simulink model "SVM_test2"  (R2020a)
(part 4 of 9)

      mask init:
      | % blkh = gcbh;
      | % [sfi, sfp, sfpt] = rti_fpga_blockinitial(blkh,'UPDATEPARAMETER');
      | % rti_fpga_blockinitial(blkh,'UPDATEBLOCKGUI');
      settings: CopyFcn=try, rti_fpga_blk_copyfcn(gcbh); catch,errordlg({lasterr, '','Please check your RTI installation.'},['Error: ' upper(bdroot)], 'replace'); end  DeleteFcn=try, rti_fpga_blk_deletefcn(gcbh); catch,errordlg({lasterr, '','Please check your RTI installation.'},['Error: ' upper(bdroot)], 'replace'); end  ModelCloseFcn=try, rti_fpga_blk_modelclosefcn(gcbh); catch,errordlg({lasterr, '','Please check your RTI installation.'},['Error: ' upper(bdroot)], 'replace'); end  PreSaveFcn=try, rti_fpga_blk_presavefcn(gcbh); catch,errordlg({lasterr, '','Please check your RTI installation.'},['Error: ' upper(bdroot)], 'replace'); end  NameChangeFcn=try, rti_fpga_blk_namechangefcn(gcbh); catch,errordlg({lasterr, '','Please check your RTI installation.'},['Error: ' upper(bdroot)], 'replace'); end  OpenFcn=try, rti_fpga_blk_openfcn(gcbh); catch,errordlg({lasterr, '','Please check your RTI installation.'},['Error: ' upper(bdroot)], 'replace'); end  CloseFcn=try, rti_fpga_blk_closefcn(gcbh); catch,errordlg({lasterr, '','Please check your RTI installation.'},['Error: ' upper(bdroot)], 'replace'); end  ParentCloseFcn=try, rti_fpga_blk_parentclosefcn(gcbh); catch,errordlg({lasterr, '','Please check your RTI installation.'},['Error: ' upper(bdroot)], 'replace'); end
      mask Help: eval( ['lasterror(''reset''); rtifpgaguilib(''RTIMaskHelp'', gcbh);', 'disp(lasterr);']);
      mask Display: text(0.5,0.65,'Register In 3','HorizontalAlignment','center');text(0.5,0.5,'cl','HorizontalAlignment','center');text(0.5,0.35,'Group: 1','HorizontalAlignment','center');
  FPGA_XDATA_READ_BL4 : Subsystem  LoadFcn=try, rti_fpga_blk_loadfcn(gcbh); catch,errordlg({lasterr, '','Please check your RTI installation.'},['Error: ' upper(bdroot)], 'replace'); end  InitFcn=try, rti_fpga_blk_initfcn(gcbh); catch,errordlg({lasterr, '','Please check your RTI installation.'},['Error: ' upper(bdroot)], 'replace'); end  StartFcn=try, rti_fpga_blk_startfcn(gcbh); catch,errordlg({lasterr, '','Please check your RTI installation.'},['Error: ' upper(bdroot)], 'replace'); end  mask(RTI){DSProperties=struct('RTI',struct('Version',uint32(6),'BlockType',struct('isSLSource',uint8(1),'isSLSink',uint8(0),'isHWSource',uint8(0),'isHWSink',uint8(0),'isSetup',uint8(1),'isInline',uint8(1),'isNonInline',uint8(0),'isInterrupt',uint8(0),'isChannelwise',uint8(0)),'IOBoardType','DSFPGA','UnitType','','Identifier','PHSREAD','DialogType','ML','BlockSet','FPGA','SlaveProcessor','')), RTIBlockInterface=struct('OutputPortsActive',1,'OutputPortsWidth',int32(1),'OutputPortsDataType',{{'SS_DOUBLE'}},'OutputPortsName',{{['From XDATA']}},'InitLevel',3,'DialogFcn','rtifpgaphsreadgui','BlockDisplay',{{['XDATA Read'],'auto'}},'IconTransparency','on','BlockName',struct('Token',{{'FPGA_XDATA_Read_BL1'}})), RTIBlockParameters=struct('BoardNo',{{1,'OFF',[1 16]}},'Name',{{['Register In 4'],'OFF',[]}},'CustomName',{{'d1','OFF',[]}},'AccessTyp',{{'Register','OFF',[]}},'ChannelNo',{{'4','OFF',[]}},'FrmIni',{{'fpga_framework_ini_DS1302_XC7K325T_FLEXIBLEIO','OFF',[]}},'DynFcn',{{struct('GUIPar',struct('Name',{{['Binary point position (or fraction width)']},{'Format'},{['Register Group ID']},{['Enable simulation port']},{['Simulation ports sample time']},{['Used Flag']}},'GUIType',{{'edit'},{'popup','signed','unsigned','floating-point'},{'edit'},{'checkbox'},{'edit'},{'none'}},'Range',{{[0 1 2 3 4 5 6 7 8 9 10 11 12 13 14 15 16 17 18 19 20 21 22 23 24 25 26 27 28 29 30 31 32]},{'signed','unsigned','floating-point'},{[0 1 2 3 4 5 6 7 8 9 10 11 12 13 14 15 16 17 18 19 20 21 22 23 24 25 26 27 28 29 30 31 32 33 34 35 36 37 38 39 40 41 42 43 44 45 46 47 48 49 50 51 52 53 54 55 56 57 58 59 60 61 62 63]},{'0','1'},{''},{'0','1'}},'Init',{{'0'},{'signed'},{'0'},{'0'},{'-1','1'},{'1','0'}},'Group',{{''},{''},{''},{''},{''},{''}},'Generic',{{''},{''},{'xreg2fpga_group_003'},{''},{'REGISTER_IN_003_SIM_PORT_SAMPLE_TIME'},{'xreg2fpga_inst_003'}},'Application',{{''},{''},{''},{'ApplicationOut(1).Show'},{''},{''}},'Framework',{{'FrameworkIn(1).BinaryPoint'},{'FrameworkIn(1).Format'},{''},{''},{''},{''}},'Callback',{{'proc_bus_fpga_framework_ini_DS1302:fraction_width'},{'proc_bus_fpga_framework_ini_DS1302:fraction_width'},{''},{''},{''},{''}}),'Exl',{{''}},'HlpFile',{{'rtifpga','REGISTER_IN_DS1302'}},'Hlp',{{['Click below for further details on this I/O function.']}},'Gen',struct('name',{'','','xreg2fpga_group_003','','REGISTER_IN_003_SIM_PORT_SAMPLE_TIME','xreg2fpga_inst_003'},'value',{'','','1','','-1','1'},'unusedinit',{'','','','','1','0'},'tag',{'','','','','',''},'filename',{'','','','','',''}),'Frm',struct('FrameworkOut',struct('Name',{},'BitWidth',{},'BinaryPoint',{},'Format',{}),'FrameworkIn',struct('Name',{{'xreg_003_dout'},{'xreg_003_dout_wr'}},'BitWidth',{{'32'},{'1'}},'BinaryPoint',{{'0'},{'0'}},'Format',{{'unsigned'},{'unsigned'}},'DownSample',{[],{true}})),'App',struct('ApplicationOut',struct('Name',{{'Sim_Data'}},'Show',{{0}}),'ApplicationIn',struct('Name',{{'Data'},{['Data New']}},'Show',{{true},{true}})),'Con',{{'FrameworkIn(1)','ApplicationIn(1)','FrameworkIn(2)','ApplicationIn(2)'}},'OffCon',{{'data_o','FrameworkIn(1)','data_i','ApplicationOut(1)','data_new_o','FrameworkIn(2)'}},'OffModel',{{'phs_read_register'}}),'OFF',[]}},'FPGAFrameworkId',{{'8','OFF',[]}},'BusSettings',{{[' '],'OFF',[]}},'SubChannelNo',{{'1','OFF',[]}}), RTISFcnParameters=struct('BoardNo','double'), RTIBlockParaDefault=struct('BoardNo',1,'Name',[' '],'CustomName',[' '],'AccessTyp',['<not selected>'],'ChannelNo',[' '],'FrmIni',[' '],'DynFcn',struct('GUIPar','','Hlp','','HlpFile','','Frm','','Gen','','Exl','','App','','Con',''),'FPGAFrameworkId',[' '],'BusSettings',[' '],'SubChannelNo','1')}
      mask init:
      | % blkh = gcbh;
      | % [sfi, sfp, sfpt] = rti_fpga_blockinitial(blkh,'UPDATEPARAMETER');
      | % rti_fpga_blockinitial(blkh,'UPDATEBLOCKGUI');
      settings: CopyFcn=try, rti_fpga_blk_copyfcn(gcbh); catch,errordlg({lasterr, '','Please check your RTI installation.'},['Error: ' upper(bdroot)], 'replace'); end  DeleteFcn=try, rti_fpga_blk_deletefcn(gcbh); catch,errordlg({lasterr, '','Please check your RTI installation.'},['Error: ' upper(bdroot)], 'replace'); end  ModelCloseFcn=try, rti_fpga_blk_modelclosefcn(gcbh); catch,errordlg({lasterr, '','Please check your RTI installation.'},['Error: ' upper(bdroot)], 'replace'); end  PreSaveFcn=try, rti_fpga_blk_presavefcn(gcbh); catch,errordlg({lasterr, '','Please check your RTI installation.'},['Error: ' upper(bdroot)], 'replace'); end  NameChangeFcn=try, rti_fpga_blk_namechangefcn(gcbh); catch,errordlg({lasterr, '','Please check your RTI installation.'},['Error: ' upper(bdroot)], 'replace'); end  OpenFcn=try, rti_fpga_blk_openfcn(gcbh); catch,errordlg({lasterr, '','Please check your RTI installation.'},['Error: ' upper(bdroot)], 'replace'); end  CloseFcn=try, rti_fpga_blk_closefcn(gcbh); catch,errordlg({lasterr, '','Please check your RTI installation.'},['Error: ' upper(bdroot)], 'replace'); end  ParentCloseFcn=try, rti_fpga_blk_parentclosefcn(gcbh); catch,errordlg({lasterr, '','Please check your RTI installation.'},['Error: ' upper(bdroot)], 'replace'); end
      mask Help: eval( ['lasterror(''reset''); rtifpgaguilib(''RTIMaskHelp'', gcbh);', 'disp(lasterr);']);
      mask Display: text(0.5,0.65,'Register In 4','HorizontalAlignment','center');text(0.5,0.5,'d1','HorizontalAlignment','center');text(0.5,0.35,'Group: 1','HorizontalAlignment','center');
  FPGA_XDATA_READ_BL5 : Subsystem  LoadFcn=try, rti_fpga_blk_loadfcn(gcbh); catch,errordlg({lasterr, '','Please check your RTI installation.'},['Error: ' upper(bdroot)], 'replace'); end  InitFcn=try, rti_fpga_blk_initfcn(gcbh); catch,errordlg({lasterr, '','Please check your RTI installation.'},['Error: ' upper(bdroot)], 'replace'); end  StartFcn=try, rti_fpga_blk_startfcn(gcbh); catch,errordlg({lasterr, '','Please check your RTI installation.'},['Error: ' upper(bdroot)], 'replace'); end  mask(RTI){DSProperties=struct('RTI',struct('Version',uint32(6),'BlockType',struct('isSLSource',uint8(1),'isSLSink',uint8(0),'isHWSource',uint8(0),'isHWSink',uint8(0),'isSetup',uint8(1),'isInline',uint8(1),'isNonInline',uint8(0),'isInterrupt',uint8(0),'isChannelwise',uint8(0)),'IOBoardType','DSFPGA','UnitType','','Identifier','PHSREAD','DialogType','ML','BlockSet','FPGA','SlaveProcessor','')), RTIBlockInterface=struct('OutputPortsActive',1,'OutputPortsWidth',int32(1),'OutputPortsDataType',{{'SS_DOUBLE'}},'OutputPortsName',{{['From XDATA']}},'InitLevel',3,'DialogFcn','rtifpgaphsreadgui','BlockDisplay',{{['XDATA Read'],'auto'}},'IconTransparency','on','BlockName',struct('Token',{{'FPGA_XDATA_Read_BL1'}})), RTIBlockParameters=struct('BoardNo',{{1,'OFF',[1 16]}},'Name',{{['Register In 5'],'OFF',[]}},'CustomName',{{'d2','OFF',[]}},'AccessTyp',{{'Register','OFF',[]}},'ChannelNo',{{'5','OFF',[]}},'FrmIni',{{'fpga_framework_ini_DS1302_XC7K325T_FLEXIBLEIO','OFF',[]}},'DynFcn',{{struct('GUIPar',struct('Name',{{['Binary point position (or fraction width)']},{'Format'},{['Register Group ID']},{['Enable simulation port']},{['Simulation ports sample time']},{['Used Flag']}},'GUIType',{{'edit'},{'popup','signed','unsigned','floating-point'},{'edit'},{'checkbox'},{'edit'},{'none'}},'Range',{{[0 1 2 3 4 5 6 7 8 9 10 11 12 13 14 15 16 17 18 19 20 21 22 23 24 25 26 27 28 29 30 31 32]},{'signed','unsigned','floating-point'},{[0 1 2 3 4 5 6 7 8 9 10 11 12 13 14 15 16 17 18 19 20 21 22 23 24 25 26 27 28 29 30 31 32 33 34 35 36 37 38 39 40 41 42 43 44 45 46 47 48 49 50 51 52 53 54 55 56 57 58 59 60 61 62 63]},{'0','1'},{''},{'0','1'}},'Init',{{'0'},{'signed'},{'0'},{'0'},{'-1','1'},{'1','0'}},'Group',{{''},{''},{''},{''},{''},{''}},'Generic',{{''},{''},{'xreg2fpga_group_004'},{''},{'REGISTER_IN_004_SIM_PORT_SAMPLE_TIME'},{'xreg2fpga_inst_004'}},'Application',{{''},{''},{''},{'ApplicationOut(1).Show'},{''},{''}},'Framework',{{'FrameworkIn(1).BinaryPoint'},{'FrameworkIn(1).Format'},{''},{''},{''},{''}},'Callback',{{'proc_bus_fpga_framework_ini_DS1302:fraction_width'},{'proc_bus_fpga_framework_ini_DS1302:fraction_width'},{''},{''},{''},{''}}),'Exl',{{''}},'HlpFile',{{'rtifpga','REGISTER_IN_DS1302'}},'Hlp',{{['Click below for further details on this I/O function.']}},'Gen',struct('name',{'','','xreg2fpga_group_004','','REGISTER_IN_004_SIM_PORT_SAMPLE_TIME','xreg2fpga_inst_004'},'value',{'','','1','','-1','1'},'unusedinit',{'','','','','1','0'},'tag',{'','','','','',''},'filename',{'','','','','',''}),'Frm',struct('FrameworkOut',struct('Name',{},'BitWidth',{},'BinaryPoint',{},'Format',{}),'FrameworkIn',struct('Name',{{'xreg_004_dout'},{'xreg_004_dout_wr'}},'BitWidth',{{'32'},{'1'}},'BinaryPoint',{{'0'},{'0'}},'Format',{{'unsigned'},{'unsigned'}},'DownSample',{[],{true}})),'App',struct('ApplicationOut',struct('Name',{{'Sim_Data'}},'Show',{{0}}),'ApplicationIn',struct('Name',{{'Data'},{['Data New']}},'Show',{{true},{true}})),'Con',{{'FrameworkIn(1)','ApplicationIn(1)','FrameworkIn(2)','ApplicationIn(2)'}},'OffCon',{{'data_o','FrameworkIn(1)','data_i','ApplicationOut(1)','data_new_o','FrameworkIn(2)'}},'OffModel',{{'phs_read_register'}}),'OFF',[]}},'FPGAFrameworkId',{{'8','OFF',[]}},'BusSettings',{{[' '],'OFF',[]}},'SubChannelNo',{{'1','OFF',[]}}), RTISFcnParameters=struct('BoardNo','double'), RTIBlockParaDefault=struct('BoardNo',1,'Name',[' '],'CustomName',[' '],'AccessTyp',['<not selected>'],'ChannelNo',[' '],'FrmIni',[' '],'DynFcn',struct('GUIPar','','Hlp','','HlpFile','','Frm','','Gen','','Exl','','App','','Con',''),'FPGAFrameworkId',[' '],'BusSettings',[' '],'SubChannelNo','1')}
      mask init:
      | % blkh = gcbh;
      | % [sfi, sfp, sfpt] = rti_fpga_blockinitial(blkh,'UPDATEPARAMETER');
      | % rti_fpga_blockinitial(blkh,'UPDATEBLOCKGUI');
      settings: CopyFcn=try, rti_fpga_blk_copyfcn(gcbh); catch,errordlg({lasterr, '','Please check your RTI installation.'},['Error: ' upper(bdroot)], 'replace'); end  DeleteFcn=try, rti_fpga_blk_deletefcn(gcbh); catch,errordlg({lasterr, '','Please check your RTI installation.'},['Error: ' upper(bdroot)], 'replace'); end  ModelCloseFcn=try, rti_fpga_blk_modelclosefcn(gcbh); catch,errordlg({lasterr, '','Please check your RTI installation.'},['Error: ' upper(bdroot)], 'replace'); end  PreSaveFcn=try, rti_fpga_blk_presavefcn(gcbh); catch,errordlg({lasterr, '','Please check your RTI installation.'},['Error: ' upper(bdroot)], 'replace'); end  NameChangeFcn=try, rti_fpga_blk_namechangefcn(gcbh); catch,errordlg({lasterr, '','Please check your RTI installation.'},['Error: ' upper(bdroot)], 'replace'); end  OpenFcn=try, rti_fpga_blk_openfcn(gcbh); catch,errordlg({lasterr, '','Please check your RTI installation.'},['Error: ' upper(bdroot)], 'replace'); end  CloseFcn=try, rti_fpga_blk_closefcn(gcbh); catch,errordlg({lasterr, '','Please check your RTI installation.'},['Error: ' upper(bdroot)], 'replace'); end  ParentCloseFcn=try, rti_fpga_blk_parentclosefcn(gcbh); catch,errordlg({lasterr, '','Please check your RTI installation.'},['Error: ' upper(bdroot)], 'replace'); end
      mask Help: eval( ['lasterror(''reset''); rtifpgaguilib(''RTIMaskHelp'', gcbh);', 'disp(lasterr);']);
      mask Display: text(0.5,0.65,'Register In 5','HorizontalAlignment','center');text(0.5,0.5,'d2','HorizontalAlignment','center');text(0.5,0.35,'Group: 1','HorizontalAlignment','center');
  FPGA_XDATA_READ_BL6 : Subsystem  LoadFcn=try, rti_fpga_blk_loadfcn(gcbh); catch,errordlg({lasterr, '','Please check your RTI installation.'},['Error: ' upper(bdroot)], 'replace'); end  InitFcn=try, rti_fpga_blk_initfcn(gcbh); catch,errordlg({lasterr, '','Please check your RTI installation.'},['Error: ' upper(bdroot)], 'replace'); end  StartFcn=try, rti_fpga_blk_startfcn(gcbh); catch,errordlg({lasterr, '','Please check your RTI installation.'},['Error: ' upper(bdroot)], 'replace'); end  mask(RTI){DSProperties=struct('RTI',struct('Version',uint32(6),'BlockType',struct('isSLSource',uint8(1),'isSLSink',uint8(0),'isHWSource',uint8(0),'isHWSink',uint8(0),'isSetup',uint8(1),'isInline',uint8(1),'isNonInline',uint8(0),'isInterrupt',uint8(0),'isChannelwise',uint8(0)),'IOBoardType','DSFPGA','UnitType','','Identifier','PHSREAD','DialogType','ML','BlockSet','FPGA','SlaveProcessor','')), RTIBlockInterface=struct('OutputPortsActive',1,'OutputPortsWidth',int32(1),'OutputPortsDataType',{{'SS_DOUBLE'}},'OutputPortsName',{{['From XDATA']}},'InitLevel',3,'DialogFcn','rtifpgaphsreadgui','BlockDisplay',{{['XDATA Read'],'auto'}},'IconTransparency','on','BlockName',struct('Token',{{'FPGA_XDATA_Read_BL1'}})), RTIBlockParameters=struct('BoardNo',{{1,'OFF',[1 16]}},'Name',{{['Register In 6'],'OFF',[]}},'CustomName',{{'d3','OFF',[]}},'AccessTyp',{{'Register','OFF',[]}},'ChannelNo',{{'6','OFF',[]}},'FrmIni',{{'fpga_framework_ini_DS1302_XC7K325T_FLEXIBLEIO','OFF',[]}},'DynFcn',{{struct('GUIPar',struct('Name',{{['Binary point position (or fraction width)']},{'Format'},{['Register Group ID']},{['Enable simulation port']},{['Simulation ports sample time']},{['Used Flag']}},'GUIType',{{'edit'},{'popup','signed','unsigned','floating-point'},{'edit'},{'checkbox'},{'edit'},{'none'}},'Range',{{[0 1 2 3 4 5 6 7 8 9 10 11 12 13 14 15 16 17 18 19 20 21 22 23 24 25 26 27 28 29 30 31 32]},{'signed','unsigned','floating-point'},{[0 1 2 3 4 5 6 7 8 9 10 11 12 13 14 15 16 17 18 19 20 21 22 23 24 25 26 27 28 29 30 31 32 33 34 35 36 37 38 39 40 41 42 43 44 45 46 47 48 49 50 51 52 53 54 55 56 57 58 59 60 61 62 63]},{'0','1'},{''},{'0','1'}},'Init',{{'0'},{'signed'},{'0'},{'0'},{'-1','1'},{'1','0'}},'Group',{{''},{''},{''},{''},{''},{''}},'Generic',{{''},{''},{'xreg2fpga_group_005'},{''},{'REGISTER_IN_005_SIM_PORT_SAMPLE_TIME'},{'xreg2fpga_inst_005'}},'Application',{{''},{''},{''},{'ApplicationOut(1).Show'},{''},{''}},'Framework',{{'FrameworkIn(1).BinaryPoint'},{'FrameworkIn(1).Format'},{''},{''},{''},{''}},'Callback',{{'proc_bus_fpga_framework_ini_DS1302:fraction_width'},{'proc_bus_fpga_framework_ini_DS1302:fraction_width'},{''},{''},{''},{''}}),'Exl',{{''}},'HlpFile',{{'rtifpga','REGISTER_IN_DS1302'}},'Hlp',{{['Click below for further details on this I/O function.']}},'Gen',struct('name',{'','','xreg2fpga_group_005','','REGISTER_IN_005_SIM_PORT_SAMPLE_TIME','xreg2fpga_inst_005'},'value',{'','','1','','-1','1'},'unusedinit',{'','','','','1','0'},'tag',{'','','','','',''},'filename',{'','','','','',''}),'Frm',struct('FrameworkOut',struct('Name',{},'BitWidth',{},'BinaryPoint',{},'Format',{}),'FrameworkIn',struct('Name',{{'xreg_005_dout'},{'xreg_005_dout_wr'}},'BitWidth',{{'32'},{'1'}},'BinaryPoint',{{'0'},{'0'}},'Format',{{'unsigned'},{'unsigned'}},'DownSample',{[],{true}})),'App',struct('ApplicationOut',struct('Name',{{'Sim_Data'}},'Show',{{0}}),'ApplicationIn',struct('Name',{{'Data'},{['Data New']}},'Show',{{true},{true}})),'Con',{{'FrameworkIn(1)','ApplicationIn(1)','FrameworkIn(2)','ApplicationIn(2)'}},'OffCon',{{'data_o','FrameworkIn(1)','data_i','ApplicationOut(1)','data_new_o','FrameworkIn(2)'}},'OffModel',{{'phs_read_register'}}),'OFF',[]}},'FPGAFrameworkId',{{'8','OFF',[]}},'BusSettings',{{[' '],'OFF',[]}},'SubChannelNo',{{'1','OFF',[]}}), RTISFcnParameters=struct('BoardNo','double'), RTIBlockParaDefault=struct('BoardNo',1,'Name',[' '],'CustomName',[' '],'AccessTyp',['<not selected>'],'ChannelNo',[' '],'FrmIni',[' '],'DynFcn',struct('GUIPar','','Hlp','','HlpFile','','Frm','','Gen','','Exl','','App','','Con',''),'FPGAFrameworkId',[' '],'BusSettings',[' '],'SubChannelNo','1')}
      mask init:
      | % blkh = gcbh;
      | % [sfi, sfp, sfpt] = rti_fpga_blockinitial(blkh,'UPDATEPARAMETER');
      | % rti_fpga_blockinitial(blkh,'UPDATEBLOCKGUI');
      settings: CopyFcn=try, rti_fpga_blk_copyfcn(gcbh); catch,errordlg({lasterr, '','Please check your RTI installation.'},['Error: ' upper(bdroot)], 'replace'); end  DeleteFcn=try, rti_fpga_blk_deletefcn(gcbh); catch,errordlg({lasterr, '','Please check your RTI installation.'},['Error: ' upper(bdroot)], 'replace'); end  ModelCloseFcn=try, rti_fpga_blk_modelclosefcn(gcbh); catch,errordlg({lasterr, '','Please check your RTI installation.'},['Error: ' upper(bdroot)], 'replace'); end  PreSaveFcn=try, rti_fpga_blk_presavefcn(gcbh); catch,errordlg({lasterr, '','Please check your RTI installation.'},['Error: ' upper(bdroot)], 'replace'); end  NameChangeFcn=try, rti_fpga_blk_namechangefcn(gcbh); catch,errordlg({lasterr, '','Please check your RTI installation.'},['Error: ' upper(bdroot)], 'replace'); end  OpenFcn=try, rti_fpga_blk_openfcn(gcbh); catch,errordlg({lasterr, '','Please check your RTI installation.'},['Error: ' upper(bdroot)], 'replace'); end  CloseFcn=try, rti_fpga_blk_closefcn(gcbh); catch,errordlg({lasterr, '','Please check your RTI installation.'},['Error: ' upper(bdroot)], 'replace'); end  ParentCloseFcn=try, rti_fpga_blk_parentclosefcn(gcbh); catch,errordlg({lasterr, '','Please check your RTI installation.'},['Error: ' upper(bdroot)], 'replace'); end
      mask Help: eval( ['lasterror(''reset''); rtifpgaguilib(''RTIMaskHelp'', gcbh);', 'disp(lasterr);']);
      mask Display: text(0.5,0.65,'Register In 6','HorizontalAlignment','center');text(0.5,0.5,'d3','HorizontalAlignment','center');text(0.5,0.35,'Group: 1','HorizontalAlignment','center');
  FPGA_XDATA_READ_BL7 : Subsystem  LoadFcn=try, rti_fpga_blk_loadfcn(gcbh); catch,errordlg({lasterr, '','Please check your RTI installation.'},['Error: ' upper(bdroot)], 'replace'); end  InitFcn=try, rti_fpga_blk_initfcn(gcbh); catch,errordlg({lasterr, '','Please check your RTI installation.'},['Error: ' upper(bdroot)], 'replace'); end  StartFcn=try, rti_fpga_blk_startfcn(gcbh); catch,errordlg({lasterr, '','Please check your RTI installation.'},['Error: ' upper(bdroot)], 'replace'); end  mask(RTI){DSProperties=struct('RTI',struct('Version',uint32(6),'BlockType',struct('isSLSource',uint8(1),'isSLSink',uint8(0),'isHWSource',uint8(0),'isHWSink',uint8(0),'isSetup',uint8(1),'isInline',uint8(1),'isNonInline',uint8(0),'isInterrupt',uint8(0),'isChannelwise',uint8(0)),'IOBoardType','DSFPGA','UnitType','','Identifier','PHSREAD','DialogType','ML','BlockSet','FPGA','SlaveProcessor','')), RTIBlockInterface=struct('OutputPortsActive',1,'OutputPortsWidth',int32(1),'OutputPortsDataType',{{'SS_DOUBLE'}},'OutputPortsName',{{['From XDATA']}},'InitLevel',3,'DialogFcn','rtifpgaphsreadgui','BlockDisplay',{{['XDATA Read'],'auto'}},'IconTransparency','on','BlockName',struct('Token',{{'FPGA_XDATA_Read_BL1'}})), RTIBlockParameters=struct('BoardNo',{{1,'OFF',[1 16]}},'Name',{{['Register In 7'],'OFF',[]}},'CustomName',{{'d4','OFF',[]}},'AccessTyp',{{'Register','OFF',[]}},'ChannelNo',{{'7','OFF',[]}},'FrmIni',{{'fpga_framework_ini_DS1302_XC7K325T_FLEXIBLEIO','OFF',[]}},'DynFcn',{{struct('GUIPar',struct('Name',{{['Binary point position (or fraction width)']},{'Format'},{['Register Group ID']},{['Enable simulation port']},{['Simulation ports sample time']},{['Used Flag']}},'GUIType',{{'edit'},{'popup','signed','unsigned','floating-point'},{'edit'},{'checkbox'},{'edit'},{'none'}},'Range',{{[0 1 2 3 4 5 6 7 8 9 10 11 12 13 14 15 16 17 18 19 20 21 22 23 24 25 26 27 28 29 30 31 32]},{'signed','unsigned','floating-point'},{[0 1 2 3 4 5 6 7 8 9 10 11 12 13 14 15 16 17 18 19 20 21 22 23 24 25 26 27 28 29 30 31 32 33 34 35 36 37 38 39 40 41 42 43 44 45 46 47 48 49 50 51 52 53 54 55 56 57 58 59 60 61 62 63]},{'0','1'},{''},{'0','1'}},'Init',{{'0'},{'signed'},{'0'},{'0'},{'-1','1'},{'1','0'}},'Group',{{''},{''},{''},{''},{''},{''}},'Generic',{{''},{''},{'xreg2fpga_group_006'},{''},{'REGISTER_IN_006_SIM_PORT_SAMPLE_TIME'},{'xreg2fpga_inst_006'}},'Application',{{''},{''},{''},{'ApplicationOut(1).Show'},{''},{''}},'Framework',{{'FrameworkIn(1).BinaryPoint'},{'FrameworkIn(1).Format'},{''},{''},{''},{''}},'Callback',{{'proc_bus_fpga_framework_ini_DS1302:fraction_width'},{'proc_bus_fpga_framework_ini_DS1302:fraction_width'},{''},{''},{''},{''}}),'Exl',{{''}},'HlpFile',{{'rtifpga','REGISTER_IN_DS1302'}},'Hlp',{{['Click below for further details on this I/O function.']}},'Gen',struct('name',{'','','xreg2fpga_group_006','','REGISTER_IN_006_SIM_PORT_SAMPLE_TIME','xreg2fpga_inst_006'},'value',{'','','1','','-1','1'},'unusedinit',{'','','','','1','0'},'tag',{'','','','','',''},'filename',{'','','','','',''}),'Frm',struct('FrameworkOut',struct('Name',{},'BitWidth',{},'BinaryPoint',{},'Format',{}),'FrameworkIn',struct('Name',{{'xreg_006_dout'},{'xreg_006_dout_wr'}},'BitWidth',{{'32'},{'1'}},'BinaryPoint',{{'0'},{'0'}},'Format',{{'unsigned'},{'unsigned'}},'DownSample',{[],{true}})),'App',struct('ApplicationOut',struct('Name',{{'Sim_Data'}},'Show',{{0}}),'ApplicationIn',struct('Name',{{'Data'},{['Data New']}},'Show',{{true},{true}})),'Con',{{'FrameworkIn(1)','ApplicationIn(1)','FrameworkIn(2)','ApplicationIn(2)'}},'OffCon',{{'data_o','FrameworkIn(1)','data_i','ApplicationOut(1)','data_new_o','FrameworkIn(2)'}},'OffModel',{{'phs_read_register'}}),'OFF',[]}},'FPGAFrameworkId',{{'8','OFF',[]}},'BusSettings',{{[' '],'OFF',[]}},'SubChannelNo',{{'1','OFF',[]}}), RTISFcnParameters=struct('BoardNo','double'), RTIBlockParaDefault=struct('BoardNo',1,'Name',[' '],'CustomName',[' '],'AccessTyp',['<not selected>'],'ChannelNo',[' '],'FrmIni',[' '],'DynFcn',struct('GUIPar','','Hlp','','HlpFile','','Frm','','Gen','','Exl','','App','','Con',''),'FPGAFrameworkId',[' '],'BusSettings',[' '],'SubChannelNo','1')}
      mask init:
      | % blkh = gcbh;
      | % [sfi, sfp, sfpt] = rti_fpga_blockinitial(blkh,'UPDATEPARAMETER');
      | % rti_fpga_blockinitial(blkh,'UPDATEBLOCKGUI');
      settings: CopyFcn=try, rti_fpga_blk_copyfcn(gcbh); catch,errordlg({lasterr, '','Please check your RTI installation.'},['Error: ' upper(bdroot)], 'replace'); end  DeleteFcn=try, rti_fpga_blk_deletefcn(gcbh); catch,errordlg({lasterr, '','Please check your RTI installation.'},['Error: ' upper(bdroot)], 'replace'); end  ModelCloseFcn=try, rti_fpga_blk_modelclosefcn(gcbh); catch,errordlg({lasterr, '','Please check your RTI installation.'},['Error: ' upper(bdroot)], 'replace'); end  PreSaveFcn=try, rti_fpga_blk_presavefcn(gcbh); catch,errordlg({lasterr, '','Please check your RTI installation.'},['Error: ' upper(bdroot)], 'replace'); end  NameChangeFcn=try, rti_fpga_blk_namechangefcn(gcbh); catch,errordlg({lasterr, '','Please check your RTI installation.'},['Error: ' upper(bdroot)], 'replace'); end  OpenFcn=try, rti_fpga_blk_openfcn(gcbh); catch,errordlg({lasterr, '','Please check your RTI installation.'},['Error: ' upper(bdroot)], 'replace'); end  CloseFcn=try, rti_fpga_blk_closefcn(gcbh); catch,errordlg({lasterr, '','Please check your RTI installation.'},['Error: ' upper(bdroot)], 'replace'); end  ParentCloseFcn=try, rti_fpga_blk_parentclosefcn(gcbh); catch,errordlg({lasterr, '','Please check your RTI installation.'},['Error: ' upper(bdroot)], 'replace'); end
      mask Help: eval( ['lasterror(''reset''); rtifpgaguilib(''RTIMaskHelp'', gcbh);', 'disp(lasterr);']);
      mask Display: text(0.5,0.65,'Register In 7','HorizontalAlignment','center');text(0.5,0.5,'d4','HorizontalAlignment','center');text(0.5,0.35,'Group: 1','HorizontalAlignment','center');
  Terminator{1..20,22..26} (25 alike) : Terminator
  wires:
  Convert1/1 -> Black Box/7
  Convert/1 -> Black Box/6
  Convert3/1 -> Black Box/5
  Convert7/1 -> Black Box/4
  Convert6/1 -> Black Box/3
  Convert5/1 -> Black Box/2
  Convert4/1 -> Black Box/1
  FPGA_XDATA_READ_BL4/2(Data New) -> Terminator23/1
  FPGA_XDATA_READ_BL1/1(Data) -> Convert3/1
  FPGA_XDATA_READ_BL2/1(Data) -> Convert/1
  FPGA_XDATA_READ_BL2/2(Data New) -> Terminator1/1
  FPGA_XDATA_READ_BL5/1(Data) -> Convert5/1
  FPGA_XDATA_READ_BL4/1(Data) -> Convert4/1
  FPGA_XDATA_READ_BL3/2(Data New) -> Terminator20/1
  FPGA_XDATA_READ_BL1/2(Data New) -> Terminator22/1
  FPGA_XDATA_READ_BL5/2(Data New) -> Terminator24/1
  FPGA_XDATA_READ_BL6/2(Data New) -> Terminator25/1
  FPGA_XDATA_READ_BL7/2(Data New) -> Terminator26/1
  FPGA_XDATA_READ_BL6/1(Data) -> Convert6/1
  FPGA_XDATA_READ_BL7/1(Data) -> Convert7/1
  FPGA_XDATA_READ_BL3/1(Data) -> Convert1/1
  FPGA_IO_WRITE_BL5/1(Data In) -> Terminator6/1
  FPGA_IO_WRITE_BL17/1(Data In) -> Terminator18/1
  FPGA_IO_WRITE_BL8/1(Data In) -> Terminator9/1
  Black Box/17 -> FPGA_IO_WRITE_BL17/1(Data Out)
  Black Box/19 -> FPGA_IO_WRITE_BL19/1(Intensity Red)
  FPGA_IO_WRITE_BL14/1(Data In) -> Terminator15/1
  Black Box/3 -> FPGA_IO_WRITE_BL3/1(Data Out)
  Constant1/1 -> FPGA_IO_WRITE_BL1/2(Enable), FPGA_IO_WRITE_BL2/2(Enable), FPGA_IO_WRITE_BL3/2(Enable), FPGA_IO_WRITE_BL4/2(Enable), FPGA_IO_WRITE_BL5/2(Enable), FPGA_IO_WRITE_BL6/2(Enable), FPGA_IO_WRITE_BL18/2(Enable), FPGA_IO_WRITE_BL17/2(Enable), FPGA_IO_WRITE_BL16/2(Enable), FPGA_IO_WRITE_BL15/2(Enable), FPGA_IO_WRITE_BL14/2(Enable), FPGA_IO_WRITE_BL13/2(Enable), FPGA_IO_WRITE_BL12/2(Enable), FPGA_IO_WRITE_BL11/2(Enable), FPGA_IO_WRITE_BL10/2(Enable), FPGA_IO_WRITE_BL9/2(Enable), FPGA_IO_WRITE_BL8/2(Enable), FPGA_IO_WRITE_BL7/2(Enable)
  Black Box/6 -> FPGA_IO_WRITE_BL6/1(Data Out)
  Black Box/4 -> FPGA_IO_WRITE_BL4/1(Data Out)
  Constant2/1 -> FPGA_IO_WRITE_BL5/3(Direction), FPGA_IO_WRITE_BL4/3(Direction), FPGA_IO_WRITE_BL1/3(Direction), FPGA_IO_WRITE_BL2/3(Direction), FPGA_IO_WRITE_BL3/3(Direction), FPGA_IO_WRITE_BL6/3(Direction), FPGA_IO_WRITE_BL7/3(Direction), FPGA_IO_WRITE_BL8/3(Direction), FPGA_IO_WRITE_BL9/3(Direction), FPGA_IO_WRITE_BL10/3(Direction), FPGA_IO_WRITE_BL11/3(Direction), FPGA_IO_WRITE_BL12/3(Direction), FPGA_IO_WRITE_BL13/3(Direction), FPGA_IO_WRITE_BL14/3(Direction), FPGA_IO_WRITE_BL15/3(Direction), FPGA_IO_WRITE_BL16/3(Direction), FPGA_IO_WRITE_BL17/3(Direction), FPGA_IO_WRITE_BL18/3(Direction)
  FPGA_IO_WRITE_BL2/1(Data In) -> Terminator3/1
  Black Box/8 -> FPGA_IO_WRITE_BL8/1(Data Out)
  FPGA_IO_WRITE_BL12/1(Data In) -> Terminator13/1
  Black Box/5 -> FPGA_IO_WRITE_BL5/1(Data Out)
  Black Box/1 -> FPGA_IO_WRITE_BL1/1(Data Out)
  FPGA_IO_WRITE_BL4/1(Data In) -> Terminator5/1
  FPGA_IO_WRITE_BL1/1(Data In) -> Terminator2/1
  Black Box/7 -> FPGA_IO_WRITE_BL7/1(Data Out)
  FPGA_IO_WRITE_BL11/1(Data In) -> Terminator12/1
  Black Box/12 -> FPGA_IO_WRITE_BL12/1(Data Out)
  Black Box/13 -> FPGA_IO_WRITE_BL13/1(Data Out)
  FPGA_IO_WRITE_BL15/1(Data In) -> Terminator16/1
  Black Box/16 -> FPGA_IO_WRITE_BL16/1(Data Out)
  FPGA_IO_WRITE_BL13/1(Data In) -> Terminator14/1
  Black Box/20 -> FPGA_IO_WRITE_BL19/2(Intensity Green)
  Black Box/22 -> FPGA_INT_BL1/1(Int)  "interr"
  Black Box/11 -> FPGA_IO_WRITE_BL11/1(Data Out)
  FPGA_IO_WRITE_BL10/1(Data In) -> Terminator11/1
  FPGA_IO_WRITE_BL7/1(Data In) -> Terminator8/1
  Black Box/15 -> FPGA_IO_WRITE_BL15/1(Data Out)
  Black Box/21 -> FPGA_IO_WRITE_BL19/3(Intensity Blue)
  FPGA_IO_WRITE_BL3/1(Data In) -> Terminator4/1
  FPGA_IO_WRITE_BL16/1(Data In) -> Terminator17/1
  Black Box/14 -> FPGA_IO_WRITE_BL14/1(Data Out)
  Black Box/10 -> FPGA_IO_WRITE_BL10/1(Data Out)
  Black Box/2 -> FPGA_IO_WRITE_BL2/1(Data Out)
  Black Box/9 -> FPGA_IO_WRITE_BL9/1(Data Out)
  Black Box/18 -> FPGA_IO_WRITE_BL18/1(Data Out)
  FPGA_IO_WRITE_BL9/1(Data In) -> Terminator10/1
  FPGA_IO_WRITE_BL6/1(Data In) -> Terminator7/1
  FPGA_IO_WRITE_BL18/1(Data In) -> Terminator19/1
  Black Box/23 -> FPGA_INT_BL2/1(Int)
